simulink model "ofdm_gito"  (Simulink 5.0)
settings: Solver=ode45  StartTime=0.0  StopTime=10.0  RelTol=1e-3
undefined symbols (not defined in the file or in its folder): Fs, rsgenpoly
libraries: dspsigattribs x6, commdigbbndpm2 x6, commsink2 x4, simulink x4, dspindex x4, commchan2 x2, dspsnks4 x2, dspxfrm3 x2, commblkcod2 x2, commseqgen2 x2, commutil2 x2, dspbuff3 x2
Description:
  | This COFDM Simulation simulate Coded OFDM using
  | Reed-Solomon Channel Coding, over wireless multipath
  | fading channel, with 3 us maximal delay spread, 200 Hz
  | Doppler shift.
  | In this simulation I use QPSK, and Training Based
  | Channel Estimation, 11/15 RS Code, 2 Symbol Error
  | Correction
  | 
  | I also have paper that report this simulation in
  | Matlab Central
  | 
  | If you interest about this simulation, please mail to
  | gito_pras@telkom.net
settings Model: Creator=Gito Prastomo  LastModifiedBy=Gito Prastomo

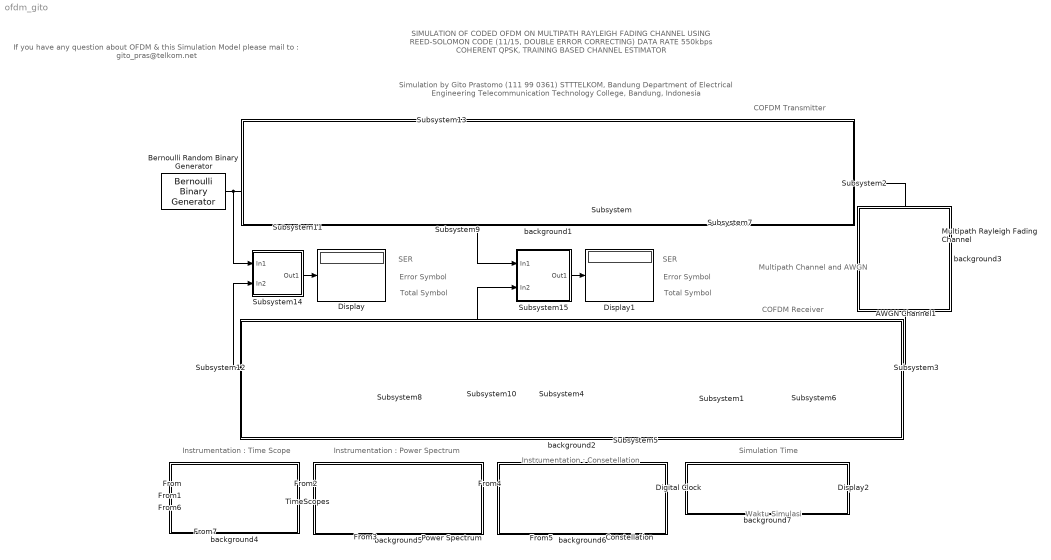
== system ofdm_gito ==
  note: SIMULATION OF CODED OFDM ON MULTIPATH RAYLEIGH FADING CHANNEL
      | USING REED-SOLOMON CODE (11/15, DOUBLE ERROR CORRECTING)
      | DATA RATE 550kbps COHERENT  QPSK, TRAINING BASED CHANNEL ESTIMATOR
  note: Simulation by Gito Prastomo (111 99 0361)
      | STTTELKOM, Bandung
      | Department of Electrical Engineering
      | Telecommunication Technology College, Bandung, Indonesia
  note: SER
  note: Error Symbol
  note: Total Symbol
  note: SER
  note: Error Symbol
  note: Total Symbol
  note: Instrumentation : Time Scope
  note: COFDM Transmitter
  note: COFDM Receiver
  note: Multipath Channel
      | and AWGN
  note: Waktu Simulasi
  note: Instrumentation : Power Spectrum
  note: Instrumentation : Consetellation
  note: Simulation Time
  note: If you have any question
      | about OFDM & this Simulation Model
      | please mail to :
      | gito_pras@telkom.net
  AWGN Channel1 : commchan2/AWGN Channel  Orientation=down  seed=32965  noiseMode="Signal to noise ratio  (Es/No)"  EsNodB=28  SNRdB=0  Ps=30/(5.5e5*11/15*2.4)*1.08  Tsym=80e-6  variance=1
  Bernoulli Random Binary Generator : commrandsrc2/Bernoulli Binary Generator  P=[0.5]  seed=9364248  Ts=16e-5/44/2  frameBased=on  sampPerFrame=44  orient=off
  Constellation : Subsystem  TreatAsAtomicUnit=on  mask(Instrumentation: Power Spectrum){On=off, Off=on}
      mask init:
      | if strcmp(On,'on')
      |   [picture, map]=imread('switch_on.jpg');
      |   sdspfscope2([],[],[],'ScopeUpdate',[bdroot '/Constellation/Before Channel Estimation'],'OpenFig');
      |   sdspfscope2([],[],[],'ScopeUpdate',[bdroot '/Constellation/After Channel Estimation'],'OpenFig');
      |   set_param([bdroot '/Constellation/Before Channel Estimation'],'OpenScopeAtSimStart','on');
      |   set_param([bdroot '/Constellation/After Channel Estimation'],'OpenScopeAtSimStart','on');
      |   
      | else
      |   [picture, map]=imread('switch_off.jpg');
      |   set_param([bdroot '/Constellation/Before Channel Estimation'],'OpenScopeAtSimStart','off');
      |   set_param([bdroot '/Constellation/After Channel Estimation'],'OpenScopeAtSimStart','off');
      |   sdspfscope2([],[],[],'ScopeUpdate',[bdroot '/Constellation/Before Channel Estimation'],'CloseFig');
      |   sdspfscope2([],[],[],'ScopeUpdate',[bdroot '/Constellation/After Channel Estimation'],'CloseFig');
      |   
      | end
      settings: OpenFcn=temp=get_param(gcb,'On');set_param(gcb,'On', get_param(gcb,'Off'));set_param(gcb,'Off', temp);
      mask Display: image(picture,'center')
  Digital Clock : DigitalClock  SampleTime=8e-5
  Display : Display
  Display1 : Display
  Display2 : Display
  Multipath Rayleigh Fading Channel : commchan2/Multipath Rayleigh Fading Channel  Orientation=down  Fd=200  simTs=8e-5/180  delayVec=[0 3e-6]  gainVecdB=[0 -8]  normGain=on  Seed=936497248
  Power Spectrum : Subsystem  TreatAsAtomicUnit=on  mask(Instrumentation: Power Spectrum){On=off, Off=on}
      mask init:
      | if strcmp(On,'on')
      |   [picture, map]=imread('switch_on.jpg');
      |   set_param([gcs '/Power Spectrum/OFDM Transmitted Spectrum'],'OpenScopeAtSimStart','on');
      |   set_param([gcs '/Power Spectrum/OFDM Received Spectrum'],'OpenScopeAtSimStart','on');
      |   sdspfscope2([],[],[],'ScopeUpdate',[gcs '/Power Spectrum/OFDM Transmitted Spectrum'],'OpenFig');
      |   sdspfscope2([],[],[],'ScopeUpdate',[gcs '/Power Spectrum/OFDM Received Spectrum'],'OpenFig');
      |     
      | else
      |   [picture, map]=imread('switch_off.jpg');
      |   set_param([gcs '/Power Spectrum/OFDM Transmitted Spectrum'],'OpenScopeAtSimStart','off');
      |   set_param([gcs '/Power Spectrum/OFDM Received Spectrum'],'OpenScopeAtSimStart','off');
      |   sdspfscope2([],[],[],'ScopeUpdate',[gcs '/Power Spectrum/OFDM Transmitted Spectrum'],'CloseFig');
      |   sdspfscope2([],[],[],'ScopeUpdate',[gcs '/Power Spectrum/OFDM Received Spectrum'],'CloseFig');
      |   
      | end
      settings: OpenFcn=temp=get_param(gcb,'On');set_param(gcb,'On', get_param(gcb,'Off'));set_param(gcb,'Off', temp);
      mask Display: image(picture,'center')
  Subsystem : Subsystem
      mask Display: disp('OFDM Baseband\nModulator\ndan\nAdd Cyclic Prefix')
  Subsystem1 : Subsystem  Orientation=left
      mask Display: disp('OFDM Baseband\nDemodulator\ndan \nRemove Cyclic prefix')
  Subsystem10 : Subsystem  Orientation=left
      mask Display: disp('Remove\nZero')
  Subsystem11 : Subsystem
      mask Display: disp('RS(15,11) Encoder')
  Subsystem12 : Subsystem  Orientation=left
      mask Display: disp('RS(15,11) Decoder')
  Subsystem13 : Subsystem
      mask Display: disp('Training')
  Subsystem14 : Subsystem
      mask Display: disp('SER\nCalculation')
  Subsystem15 : Subsystem
      mask Display: disp('SER\nCalculation')
  Subsystem2 : Subsystem
      mask Display: disp('P/S')
  Subsystem3 : Subsystem  Orientation=left
      mask Display: disp('S/P')
  Subsystem4 : Subsystem  Orientation=left
      mask Display: disp('Channel\nCompensation')
  Subsystem5 : Subsystem  Orientation=left
      mask Display: disp('Channel\nEstimator')
  Subsystem6 : Subsystem  Orientation=left
      mask Display: disp('Training\nSeparation')
  Subsystem7 : Subsystem
      mask Display: disp('Training\nInsertion')
  Subsystem8 : Subsystem  Orientation=left
      mask Display: disp('QPSK Demapping')
  Subsystem9 : Subsystem
      mask Display: disp('QPSK Mapping')
  TimeScopes : Subsystem  TreatAsAtomicUnit=on  mask(Instrumentation: Power Spectrum){On=off, Off=on}
      mask init:
      | ssName=gcs;
      | if strcmp(On,'on')
      |   [picture, map]=imread('switch_on.jpg');
      |   set_param([ssName '/TimeScopes/Sinyal kirim OFDM'],'Open','on');
      |   set_param([ssName '/TimeScopes/Sinyal terima OFDM'],'Open','on');
      | else
      |     [picture, map]=imread('switch_off.jpg');
      |   set_param([ssName '/TimeScopes/Sinyal kirim OFDM'],'Open','off');
      |   set_param([ssName '/TimeScopes/Sinyal terima OFDM'],'Open','off');
      | end
      settings: OpenFcn=temp=get_param(gcb,'On');set_param(gcb,'On', get_param(gcb,'Off'));set_param(gcb,'Off', temp);
      mask Display: image(picture,'center')
  background1 : Subsystem
      mask Display: disp('')
  background2 : Subsystem
      mask Display: disp('')
  background3 : Subsystem
      mask Display: disp('')
  background4 : Subsystem
      mask Display: disp('')
  background5 : Subsystem
      mask Display: disp('')
  background6 : Subsystem
      mask Display: disp('')
  background7 : Subsystem
      mask Display: disp('')
  wires:
  Bernoulli Random Binary Generator/1 -> Subsystem11/1(In1), Subsystem14/1(In1)
  Subsystem11/1(Out1) -> Subsystem9/1(In1), Subsystem15/1(In1)
  Subsystem9/1(Out1) -> Subsystem/2(In2)
  Subsystem13/1(Out1) -> Subsystem/1(In1)
  Subsystem1/1(Out1) -> Subsystem4/1(In1)
  Subsystem1/2(Out2) -> Subsystem5/1(In1)
  Subsystem5/1(Out1) -> Subsystem4/2(In2)
  Subsystem4/1(Out1) -> Subsystem10/1(In1)
  Subsystem12/1(Out1) -> Subsystem14/2(In2)
  Subsystem8/1(Out1) -> Subsystem12/1(In1), Subsystem15/2(In2)
  Subsystem/1(Out1) -> Subsystem7/1(In1)
  Subsystem7/1(Out1) -> Subsystem2/1(In1)
  Subsystem6/1(Out1) -> Subsystem1/1(In1)
  Subsystem14/1(Out1) -> Display/1
  Subsystem3/1(Out1) -> Subsystem6/1(In1)
  Subsystem2/1(Out1) -> Multipath Rayleigh Fading Channel/1
  Subsystem10/1(Out1) -> Subsystem8/1(In1)
  Multipath Rayleigh Fading Channel/1 -> AWGN Channel1/1
  AWGN Channel1/1 -> Subsystem3/1(In1)
  Subsystem15/1(Out1) -> Display1/1
  [real_tx] -> TimeScopes/1(In1)
  [im_tx] -> TimeScopes/2(In2)
  Digital Clock/1 -> Display2/1
  [spektrum_kirim] -> Power Spectrum/1(In1)
  [spektrum_terima] -> Power Spectrum/2(In3)
  [konstelasi_sbl] -> Constellation/1(In1)
  [konstelasi_stl] -> Constellation/2(In2)
  [real_rx] -> TimeScopes/3(In3)
  [im_rx] -> TimeScopes/4(In4)

== system ofdm_gito/Constellation ==
  In1 : Inport
  In2 : Inport  Port=2
  After Channel Estimation : commsink2/Discrete-Time Scatter Plot Scope  Tag=ScatterPlot  showPlotting=on  sampPerSymb=1  offsetEye=0  numTraces=100  numNewFrames=50  showRendering=off  LineMarkers=.  LineColors=b  fading=on  render=off  AxisGrid=on  showAxes=off  xMin=-1.38590807368272  xMax=1.18815068657491  yMin=-1.28146244316  yMax=1.29259631709763  inphaseLabel=In-phase Amplitude  quadratureLabel=Quadrature Amplitude  showFigure=off  openScopeAtSimStart=off  FrameNumber=off  FigPos=[443 257 328 328]  figTitle=Scatter Plot  numLinesMax=50  block_type_=scatter
  Before Channel Estimation : commsink2/Discrete-Time Scatter Plot Scope  Tag=ScatterPlot  showPlotting=on  sampPerSymb=1  offsetEye=0  numTraces=100  numNewFrames=50  showRendering=off  LineMarkers=.  LineColors=[1 0 0]  fading=on  render=off  AxisGrid=on  showAxes=off  xMin=-3.00315520547955  xMax=2.96563413273983  yMin=-2.96784165209088  yMax=3.00094768612849  inphaseLabel=In-phase Amplitude  quadratureLabel=Quadrature Amplitude  showFigure=off  openScopeAtSimStart=off  FrameNumber=off  FigPos=[114 264 320 320]  figTitle=Scatter Plot  numLinesMax=50  block_type_=scatter
  wires:
  In1/1 -> Before Channel Estimation/1
  In2/1 -> After Channel Estimation/1

== system ofdm_gito/Power Spectrum ==
  In1 : Inport
  In3 : Inport  Port=2
  OFDM Received Spectrum : dspsnks4/Spectrum Scope  ScopeProperties=on  Domain=Frequency  HorizSpan=1  UseBuffer=on  BufferSize=90  Overlap=0  inpFftLenInherit=on  FFTlength=1024  numAvg=16  DisplayProperties=off  AxisGrid=on  Memory=off  FrameNumber=on  AxisLegend=off  AxisZoom=off  OpenScopeAtSimStart=off  OpenScopeImmediately=off  FigPos=[516 326 489 207]  AxisProperties=off  XUnits=Hertz  XRange=[-Fs/2...Fs/2]  InheritXIncr=on  XIncr=1.0  XLabel=Samples  YUnits=dB  YLabel=Magnitude, dB  LineProperties=off
      settings: YMin=-56.109120379899  YMax=-11.668971465058
  OFDM Transmitted Spectrum : dspsnks4/Spectrum Scope  ScopeProperties=on  Domain=Frequency  HorizSpan=1  UseBuffer=on  BufferSize=90  Overlap=0  inpFftLenInherit=on  FFTlength=1024  numAvg=16  DisplayProperties=off  AxisGrid=on  Memory=off  FrameNumber=on  AxisLegend=off  AxisZoom=off  OpenScopeAtSimStart=off  OpenScopeImmediately=off  FigPos=[16 327 493 204]  AxisProperties=off  XUnits=Hertz  XRange=[-Fs/2...Fs/2]  InheritXIncr=on  XIncr=1.0  XLabel=Samples  YUnits=dB  YLabel=Magnitude, dB  LineProperties=off  LineStyles=-  LineColors=[0 0 0]
      settings: YMin=-109.63726086101  YMax=-10.5147246232599
  wires:
  In3/1 -> OFDM Received Spectrum/1
  In1/1 -> OFDM Transmitted Spectrum/1

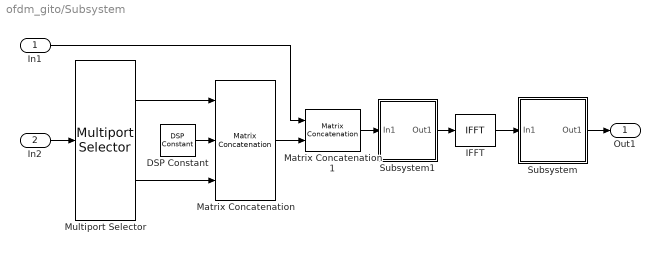
== system ofdm_gito/Subsystem ==
  In1 : Inport
  In2 : Inport  Port=2
  DSP Constant : dspsrcs4/DSP Constant  Value=0  SampleMode=Discrete  discreteOutput=Frame-based  continuousOutput=Sample-based  sampTime=16e-5/2  framePeriod=16e-5/2  dataType=Inherit from 'Constant value'  wordLen=16  udDataType=sfix(16)  fracBitsMode=Best precision  numFracBits=15  InterpretAs1D=off  Ts=16e-5/2  FramebasedOutput=on
  IFFT : dspxfrm3/IFFT  CompMethod=Table lookup  TableOpt=Speed  BitRevOrder=off  cs_in=off  SkipNorm=off  mode=Real
  Matrix Concatenation : simulink/Math Operations/Matrix Concatenation  numInports=3  catMethod=Vertical
  Matrix Concatenation1 : simulink/Math Operations/Matrix Concatenation  numInports=2  catMethod=Horizontal
  Multiport Selector : dspindex/Multiport Selector  rowsOrCols=Rows  idxCellArray={1:15,16:30}  idxErrMode=Clip Index
  Subsystem : Subsystem
      mask Display: disp('Add\nCyclic Prefix')
  Subsystem1 : Subsystem
      mask Display: disp('Zero Pad')
  Out1 : Outport
  wires:
  IFFT/1 -> Subsystem/1(In1)
  Multiport Selector/1 -> Matrix Concatenation/1
  Multiport Selector/2 -> Matrix Concatenation/3
  DSP Constant/1 -> Matrix Concatenation/2
  Subsystem1/1(Out1) -> IFFT/1
  Subsystem/1(Out1) -> Out1/1
  In2/1 -> Multiport Selector/1
  Matrix Concatenation1/1 -> Subsystem1/1(In1)
  Matrix Concatenation/1 -> Matrix Concatenation1/2
  In1/1 -> Matrix Concatenation1/1

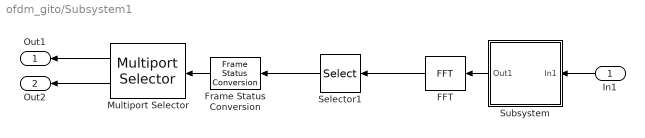
== system ofdm_gito/Subsystem1 ==
  In1 : Inport  Orientation=left
  FFT : dspxfrm3/FFT  Orientation=left  CompMethod=Table lookup  TableOpt=Speed  BitRevOrder=off
  Frame Status Conversion : dspsigattribs/Frame Status Conversion  Orientation=left  growRefPort=off  outframe=Frame-based
  Multiport Selector : dspindex/Multiport Selector  Orientation=left  rowsOrCols=Columns  idxCellArray={1,2}  idxErrMode=Clip Index
  Selector1 : Selector  Orientation=left  InputType=Matrix  Elements=[50:64,1:16]  Rows=[50:64,1:16]  Columns=-1  InputPortWidth=64
  Subsystem : Subsystem  Orientation=left
      mask Display: disp('Remove\nCyclic Prefix')
  Out1 : Outport  Orientation=left
  Out2 : Outport  Orientation=left  Port=2
  wires:
  FFT/1 -> Selector1/1
  Selector1/1 -> Frame Status Conversion/1
  Subsystem/1(Out1) -> FFT/1
  In1/1 -> Subsystem/1(In1)
  Frame Status Conversion/1 -> Multiport Selector/1
  Multiport Selector/1 -> Out1/1
  Multiport Selector/2 -> Out2/1

== system ofdm_gito/Subsystem10 ==
  In1 : Inport  Orientation=left
  Selector2 : Selector  Orientation=left  InputType=Matrix  Elements=[1:15,17:31]  Rows=[1:15,17:31]  Columns=-1  InputPortWidth=31
  Out1 : Outport  Orientation=left
  tag scope: konstelasi_stl=global
  wires:
  Selector2/1 -> Out1/1, [konstelasi_stl]
  In1/1 -> Selector2/1

== system ofdm_gito/Subsystem11 ==
  In1 : Inport
  Binary-Input RS Encoder : commblkcod2/Binary-Input RS Encoder  n=15  k=11  specPrimPoly=off  primPoly=[1 0 1 1]  specGenPoly=off  genPoly=rsgenpoly(7,3)
  Out1 : Outport
  wires:
  In1/1 -> Binary-Input RS Encoder/1
  Binary-Input RS Encoder/1 -> Out1/1

== system ofdm_gito/Subsystem12 ==
  In1 : Inport  Orientation=left
  Binary-Output RS Decoder : commblkcod2/Binary-Output RS Decoder  Orientation=left  n=15  k=11  specPrimPoly=off  primPoly=[1 0 1 1]  specGenPoly=off  genPoly=rsgenpoly(7,3)  showNumErr=on
  Terminator : Terminator
  Out1 : Outport  Orientation=left
  wires:
  Binary-Output RS Decoder/2 -> Terminator/1
  Binary-Output RS Decoder/1 -> Out1/1
  In1/1 -> Binary-Output RS Decoder/1

== system ofdm_gito/Subsystem13 ==
  PN Sequence Generator : commseqgen2/PN Sequence Generator  poly=[1 0 0 0 0 1 1]  ini_sta=[0 0 0 0 0 1]  shift=0  Ts=16e-5/2/31  frameBased=on  sampPerFrame=31  reset=off
  Unipolar to Bipolar Converter : commutil2/Unipolar to Bipolar Converter  M=2  polarity=Positive
  Out1 : Outport
  wires:
  PN Sequence Generator/1 -> Unipolar to Bipolar Converter/1
  Unipolar to Bipolar Converter/1 -> Out1/1

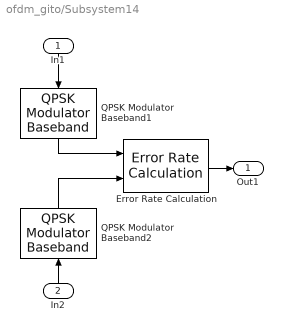
== system ofdm_gito/Subsystem14 ==
  In1 : Inport  Orientation=down
  In2 : Inport  Orientation=up  Port=2
  Error Rate Calculation : commsink2/Error Rate Calculation  N=22  st_delay=0  cp_mode=Entire frame  subframe=[]  PMode=Port  WsName=ErrorVec  RsMode2=off  stop=off  numErr=inf  maxBits=2e4
  QPSK Modulator Baseband1 : commdigbbndpm2/QPSK Modulator Baseband  Orientation=down  InType=Bit  Enc=Gray  Ph=pi/4  numSamp=1
  QPSK Modulator Baseband2 : commdigbbndpm2/QPSK Modulator Baseband  Orientation=up  InType=Bit  Enc=Gray  Ph=pi/4  numSamp=1
  Out1 : Outport
  wires:
  QPSK Modulator Baseband1/1 -> Error Rate Calculation/1
  QPSK Modulator Baseband2/1 -> Error Rate Calculation/2
  In1/1 -> QPSK Modulator Baseband1/1
  Error Rate Calculation/1 -> Out1/1
  In2/1 -> QPSK Modulator Baseband2/1

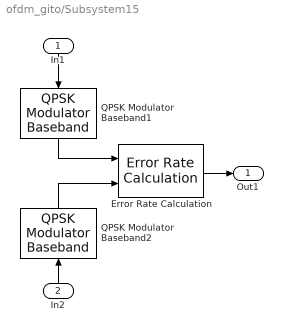
== system ofdm_gito/Subsystem15 ==
  In1 : Inport  Orientation=down
  In2 : Inport  Orientation=up  Port=2
  Error Rate Calculation : commsink2/Error Rate Calculation  N=30  st_delay=0  cp_mode=Entire frame  subframe=[]  PMode=Port  WsName=ErrorVec  RsMode2=off  stop=off  numErr=inf  maxBits=2e4
  QPSK Modulator Baseband1 : commdigbbndpm2/QPSK Modulator Baseband  Orientation=down  InType=Bit  Enc=Gray  Ph=pi/4  numSamp=1
  QPSK Modulator Baseband2 : commdigbbndpm2/QPSK Modulator Baseband  Orientation=up  InType=Bit  Enc=Gray  Ph=pi/4  numSamp=1
  Out1 : Outport
  wires:
  QPSK Modulator Baseband1/1 -> Error Rate Calculation/1
  QPSK Modulator Baseband2/1 -> Error Rate Calculation/2
  In1/1 -> QPSK Modulator Baseband1/1
  Error Rate Calculation/1 -> Out1/1
  In2/1 -> QPSK Modulator Baseband2/1

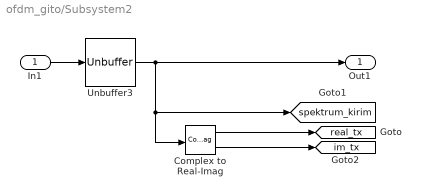
== system ofdm_gito/Subsystem2 ==
  In1 : Inport
  Complex to Real-Imag : ComplexToRealImag
  Unbuffer3 : dspbuff3/Unbuffer  ic=0
  Out1 : Outport
  tag scope: im_tx=global, real_tx=global, spektrum_kirim=global
  wires:
  In1/1 -> Unbuffer3/1
  Unbuffer3/1 -> Out1/1, Complex to Real-Imag/1, [spektrum_kirim]
  Complex to Real-Imag/1 -> [real_tx]
  Complex to Real-Imag/2 -> [im_tx]

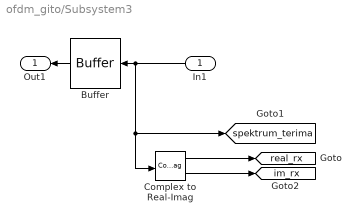
== system ofdm_gito/Subsystem3 ==
  In1 : Inport  Orientation=left
  Buffer : dspbuff3/Buffer  Orientation=left  N=180  V=0  ic=0
  Complex to Real-Imag : ComplexToRealImag
  Out1 : Outport  Orientation=left
  tag scope: im_rx=global, real_rx=global, spektrum_terima=global
  wires:
  In1/1 -> Buffer/1, [spektrum_terima], Complex to Real-Imag/1
  Buffer/1 -> Out1/1
  Complex to Real-Imag/1 -> [real_rx]
  Complex to Real-Imag/2 -> [im_rx]

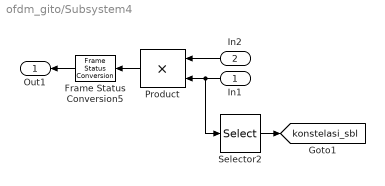
== system ofdm_gito/Subsystem4 ==
  In1 : Inport  Orientation=left
  In2 : Inport  Orientation=left  Port=2
  Frame Status Conversion5 : dspsigattribs/Frame Status Conversion  Orientation=left  growRefPort=off  outframe=Frame-based
  Product : Product  Orientation=left  SaturateOnIntegerOverflow=on
  Selector2 : Selector  InputType=Matrix  Elements=[1:15,17:31]  Rows=[1:15,17:31]  Columns=-1  InputPortWidth=31
  Out1 : Outport  Orientation=left
  tag scope: konstelasi_sbl=global
  wires:
  Product/1 -> Frame Status Conversion5/1
  Frame Status Conversion5/1 -> Out1/1
  In2/1 -> Product/1
  In1/1 -> Selector2/1, Product/2
  Selector2/1 -> [konstelasi_sbl]

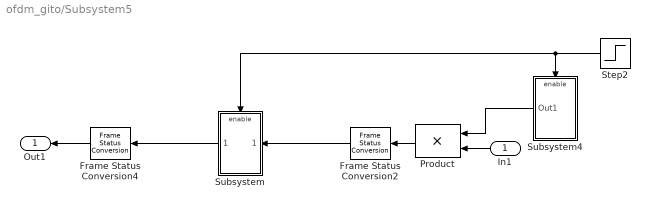
== system ofdm_gito/Subsystem5 ==
  In1 : Inport  Orientation=left
  Frame Status Conversion2 : dspsigattribs/Frame Status Conversion  Orientation=left  growRefPort=off  outframe=Frame-based
  Frame Status Conversion4 : dspsigattribs/Frame Status Conversion  Orientation=left  growRefPort=off  outframe=Frame-based
  Product : Product  Orientation=left  SaturateOnIntegerOverflow=on
  Step2 : Step  Orientation=left  Time=16e-5/2  SampleTime=16e-5/2
  Subsystem : Subsystem  Orientation=left
  Subsystem4 : Subsystem  Orientation=left  TreatAsAtomicUnit=on
  Out1 : Outport  Orientation=left
  wires:
  Step2/1 -> Subsystem4/Enable, Subsystem/Enable
  Subsystem4/1(Out1) -> Product/1
  Product/1 -> Frame Status Conversion2/1
  Frame Status Conversion2/1 -> Subsystem/1(In1)
  Frame Status Conversion4/1 -> Out1/1
  In1/1 -> Product/2
  Subsystem/1(Out1) -> Frame Status Conversion4/1

== system ofdm_gito/Subsystem6 ==
  In1 : Inport  Orientation=left
  Matrix Concatenation1 : simulink/Math Operations/Matrix Concatenation  Orientation=left  numInports=2  catMethod=Horizontal
  Multiport Selector1 : dspindex/Multiport Selector  Orientation=left  rowsOrCols=Rows  idxCellArray={91:180,1:90}  idxErrMode=Clip Index
  Out1 : Outport  Orientation=left
  wires:
  Multiport Selector1/2 -> Matrix Concatenation1/2
  Multiport Selector1/1 -> Matrix Concatenation1/1
  In1/1 -> Multiport Selector1/1
  Matrix Concatenation1/1 -> Out1/1

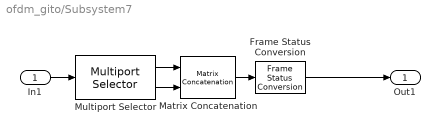
== system ofdm_gito/Subsystem7 ==
  In1 : Inport
  Frame Status Conversion : dspsigattribs/Frame Status Conversion  growRefPort=off  outframe=Frame-based
  Matrix Concatenation : simulink/Math Operations/Matrix Concatenation  numInports=2  catMethod=Vertical
  Multiport Selector : dspindex/Multiport Selector  rowsOrCols=Columns  idxCellArray={1,2}  idxErrMode=Clip Index
  Out1 : Outport
  wires:
  Multiport Selector/1 -> Matrix Concatenation/1
  Multiport Selector/2 -> Matrix Concatenation/2
  Matrix Concatenation/1 -> Frame Status Conversion/1
  In1/1 -> Multiport Selector/1
  Frame Status Conversion/1 -> Out1/1

== system ofdm_gito/Subsystem8 ==
  In1 : Inport  Orientation=left
  Gain : Gain  Orientation=left  Gain=0.75  SaturateOnIntegerOverflow=on
  QPSK Demodulator Baseband : commdigbbndpm2/QPSK Demodulator Baseband  Orientation=left  OutType=Bit  Dec=Gray  Ph=pi/4  numSamp=1
  Rounding Function : Rounding  Orientation=left  Operator=round
  Out1 : Outport  Orientation=left
  wires:
  In1/1 -> Gain/1
  Rounding Function/1 -> Out1/1
  QPSK Demodulator Baseband/1 -> Rounding Function/1
  Gain/1 -> QPSK Demodulator Baseband/1

== system ofdm_gito/Subsystem9 ==
  In1 : Inport
  Gain : Gain  Gain=1/0.75  SaturateOnIntegerOverflow=on
  QPSK Modulator Baseband : commdigbbndpm2/QPSK Modulator Baseband  InType=Bit  Enc=Gray  Ph=pi/4  numSamp=1
  Out1 : Outport
  wires:
  QPSK Modulator Baseband/1 -> Gain/1
  In1/1 -> QPSK Modulator Baseband/1
  Gain/1 -> Out1/1

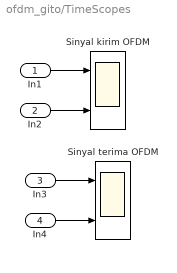
== system ofdm_gito/TimeScopes ==
  In1 : Inport
  In2 : Inport  Port=2
  In3 : Inport  Port=3
  In4 : Inport  Port=4
  Sinyal kirim OFDM : Scope  NumInputPorts=2
      settings: TimeRange=0.00030000000000008  YMin=-0.25~-0.2  YMax=0.2~0.25  SaveName=ScopeData6  DataFormat=Structure  MaxDataPoints=512
  Sinyal terima OFDM : Scope  NumInputPorts=2
      settings: TimeRange=0.00030000000000008  YMin=-0.25~-0.2  YMax=0.2~0.25  DataFormat=Structure  MaxDataPoints=512
  wires:
  In2/1 -> Sinyal kirim OFDM/2
  In1/1 -> Sinyal kirim OFDM/1
  In3/1 -> Sinyal terima OFDM/1
  In4/1 -> Sinyal terima OFDM/2

== system ofdm_gito/background1 ==

== system ofdm_gito/background2 ==

== system ofdm_gito/background3 ==

== system ofdm_gito/background4 ==

== system ofdm_gito/background5 ==

== system ofdm_gito/background6 ==

== system ofdm_gito/background7 ==

== system ofdm_gito/Subsystem/Subsystem ==
  In1 : Inport
  Selector3 : Selector  InputType=Matrix  Elements=[51:64,1:64]  Rows=[39:64,1:64]  Columns=-1  InputPortWidth=64
  Out1 : Outport
  wires:
  Selector3/1 -> Out1/1
  In1/1 -> Selector3/1

== system ofdm_gito/Subsystem/Subsystem1 ==
  In1 : Inport
  Selector : Selector  InputType=Matrix  Elements=[16:64,1:15]  Rows=[16:64,1:15]  Columns=-1  InputPortWidth=64
  Zero Pad : dspsigops/Zero Pad  padSigAt=End  zpadAlong=Columns and rows  padNumOutRowsSpecMethod=User-specified  numOutRows=64  padNumOutColsSpecMethod=User-specified  numOutCols=2  trunc_flag=None
  Out1 : Outport
  wires:
  Zero Pad/1 -> Selector/1
  In1/1 -> Zero Pad/1
  Selector/1 -> Out1/1

== system ofdm_gito/Subsystem1/Subsystem ==
  In1 : Inport  Orientation=left
  Selector4 : Selector  Orientation=left  InputType=Matrix  Elements=[15:78]  Rows=[27:90]  Columns=-1  InputPortWidth=78
  Out1 : Outport  Orientation=left
  wires:
  Selector4/1 -> Out1/1
  In1/1 -> Selector4/1

== system ofdm_gito/Subsystem5/Subsystem ==
  In1 : Inport  Orientation=left
  Enable : EnablePort
  Math Function : Math  Orientation=left  Operator=reciprocal
  Out1 : Outport  Orientation=left
  wires:
  In1/1 -> Math Function/1
  Math Function/1 -> Out1/1

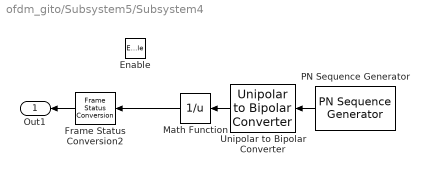
== system ofdm_gito/Subsystem5/Subsystem4 ==
  Enable : EnablePort
  Frame Status Conversion2 : dspsigattribs/Frame Status Conversion  Orientation=left  growRefPort=off  outframe=Frame-based
  Math Function : Math  Orientation=left  Operator=reciprocal
  PN Sequence Generator : commseqgen2/PN Sequence Generator  Orientation=left  poly=[1 0 0 0 0 1 1]  ini_sta=[0 0 0 0 0 1]  shift=0  Ts=16e-5/2/31  frameBased=on  sampPerFrame=31  reset=off
  Unipolar to Bipolar Converter : commutil2/Unipolar to Bipolar Converter  Orientation=left  M=2  polarity=Positive
  Out1 : Outport  Orientation=left
  wires:
  PN Sequence Generator/1 -> Unipolar to Bipolar Converter/1
  Frame Status Conversion2/1 -> Out1/1
  Math Function/1 -> Frame Status Conversion2/1
  Unipolar to Bipolar Converter/1 -> Math Function/1
